simulink model "test_R2015b"  (R2015b)
settings: Solver=VariableStepAuto  StartTime=0.0  StopTime=10.0  RelTol=1e-3
settings Model: Creator=MiaoshunWu  LastModifiedBy=MiaoshunWu

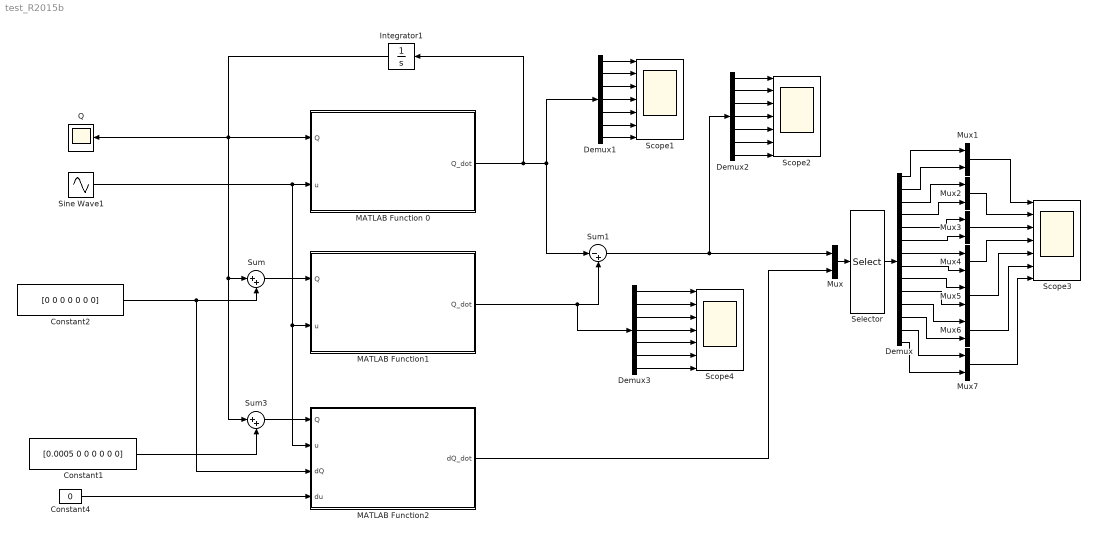
== system test_R2015b ==
  Constant1 : Constant  Value=[0.0005 0 0 0 0 0 0]
  Constant2 : Constant  Value=[0 0 0 0 0 0 0]
  Constant4 : Constant  Value=0
  Demux : Demux  Outputs=14
  Demux1 : Demux  Outputs=7
  Demux2 : Demux  Outputs=7
  Demux3 : Demux  Outputs=7
  Integrator1 : Integrator  InitialCondition=[0;0;0;0;0;0;0;]
  MATLAB Function 0 : MATLAB Function  TreatAsAtomicUnit=on
  MATLAB Function1 : MATLAB Function  TreatAsAtomicUnit=on
  MATLAB Function2 : MATLAB Function  TreatAsAtomicUnit=on
  Mux{,1..7} (8 alike) : Mux  Inputs=2
  Q : Scope
  Scope{1..4} (4 alike) : Scope  NumInputPorts=7
  Selector : Selector  InputPortWidth=14  IndexOptions=Index vector (dialog)  Indices=[1 8 2 9 3 10 4 11 5 12 6 13 7 14]  OutputSizes=1
  Sine Wave1 : Sin  SampleTime=0
  Sum : Sum  Inputs=|++
  Sum1 : Sum  Inputs=|-+
  Sum3 : Sum  Inputs=|++
  wires:
  MATLAB Function 0/1(Q_dot) -> Integrator1/1, Demux1/1, Sum1/1
  Sine Wave1/1 -> MATLAB Function 0/2(u), MATLAB Function1/2(u), MATLAB Function2/2(u)
  Sum/1 -> MATLAB Function1/1(Q)
  Integrator1/1 -> Sum3/1, Sum/1, Q/1, MATLAB Function 0/1(Q)
  MATLAB Function2/1(dQ_dot) -> Mux/2
  Constant2/1 -> MATLAB Function2/3(dQ), Sum/2
  Constant1/1 -> Sum3/2
  Sum3/1 -> MATLAB Function2/1(Q)
  Constant4/1 -> MATLAB Function2/4(du)
  Mux/1 -> Selector/1
  Selector/1 -> Demux/1
  Demux/1 -> Mux1/1
  Mux2/1 -> Scope3/2
  Mux3/1 -> Scope3/3
  Demux/7 -> Mux4/1
  Demux/8 -> Mux4/2
  Mux1/1 -> Scope3/1
  Mux4/1 -> Scope3/4
  Demux/6 -> Mux3/2
  Demux/5 -> Mux3/1
  Demux/4 -> Mux2/2
  Demux/3 -> Mux2/1
  Demux/2 -> Mux1/2
  Demux/9 -> Mux5/1
  Demux/10 -> Mux5/2
  Demux/11 -> Mux6/1
  Demux/12 -> Mux6/2
  Demux/13 -> Mux7/1
  Demux/14 -> Mux7/2
  Mux5/1 -> Scope3/5
  Mux6/1 -> Scope3/6
  Mux7/1 -> Scope3/7
  Demux1/1 -> Scope1/1
  Demux1/2 -> Scope1/2
  Demux1/3 -> Scope1/3
  Demux1/4 -> Scope1/4
  Demux1/5 -> Scope1/5
  Demux1/6 -> Scope1/6
  Demux1/7 -> Scope1/7
  Sum1/1 -> Demux2/1, Mux/1
  Demux2/1 -> Scope2/1
  Demux2/2 -> Scope2/2
  Demux2/3 -> Scope2/3
  Demux2/4 -> Scope2/4
  Demux2/5 -> Scope2/5
  Demux2/6 -> Scope2/6
  Demux2/7 -> Scope2/7
  MATLAB Function1/1(Q_dot) -> Demux3/1, Sum1/2
  Demux3/1 -> Scope4/1
  Demux3/2 -> Scope4/2
  Demux3/3 -> Scope4/3
  Demux3/4 -> Scope4/4
  Demux3/5 -> Scope4/5
  Demux3/6 -> Scope4/6
  Demux3/7 -> Scope4/7

== matlab function test_R2015b/MATLAB Function 0 ==
  data: Q_dot output; Q input; u input
function Q_dot  = DIP_Model(Q,u)
%{
%Description: Double inverted pendulum model
%Purpose: Simulates the double inverted pendulum through its mathematical 
%         dynamic model            
%Input Parameters: State space "Q", control input "u"
%Output Parameters: Derivative state space "Q_dot"
%Author: A. Arreortua
%**************************************************************************
%}
%% Definition of constants
% gravity acceleration
g = 9.81; % [m/s^2]
a1=0.085; %Distance between pivot and center of mass of pendulum1 [m]
a2=0.157; %Distance between pivot and center of mass of pendulum2 [m]
l1= 0.170; %Length of pendulum1 [m]
l2= 0.314;  %Length of pendulum2 [m]
m=0.5;  %Mass of the cart [kg]
m1=0.162; %Mass of pendulum1 [kg]
m2=0.203; %Mass of pendulum2 [kg]
J1 = (m1*l1^2)/12;    %Inertia of pendulum1 around the joint [kg m^2]
J2 = (m2*l2^2)/12;    %Inertia of pendulum2 around the joint [kg m^2]
% Model of motor behaviour: PT1 tau
T1 = 0.0395; % [s]
%Dinamic model constants
h1 = m+m1+m2;
h2 = m1*a1+m2*l1;
h3 = m2*a2;
h4 = m1*a1^2+m2*l1^2+J1;
h5 = m2*a2*l1;
h6 = m2*a2^2+J2;
h7 = m1*a1*g + m2*l1*g;
h8 = m2*a2*g;

%Q=[0;0;0;0;0;0];
det = (h4 * h6 - h5 * h5 * cos(Q(3) - Q(4)) * cos(Q(3) - Q(4)));
M11inv= [h6/det ,-h5*cos(Q(3)-Q(4))/det ; -h5*cos(Q(3)-Q(4))/det ,h4/det];
M11= [h6 ,-h5*cos(Q(3)-Q(4)) ; -h5*cos(Q(3)-Q(4)) ,h4];
M12 = [h2*cos(Q(3)); h3*cos(Q(4))];

C1 = [h5*(Q(2)^2)*sin(Q(3)-Q(4)); -h5*(Q(1)^2)*sin(Q(3)-Q(4))];
G1 = [-h7*sin(Q(3)); -h8*sin(Q(4))];
%% Dynamic equaations
x_2dot = u/T1- Q(6)/T1;  %%% x_2dot=
Theta_2dot = -M11inv*(M12* x_2dot + C1 + G1);
Q_dot = [Theta_2dot;Q(1);Q(2);Q(6);x_2dot;u*u];

== matlab function test_R2015b/MATLAB Function1 ==
  data: Q_dot output; Q input; u input
function Q_dot = DIP_Model(Q,u)
%% Definition of constants
% gravity acceleration
g = 9.81; % [m/s^2]
a1=0.085; %Distance between pivot and center of mass of pendulum1 [m]
a2=0.157; %Distance between pivot and center of mass of pendulum2 [m]
l1= 0.170; %Length of pendulum1 [m]
l2= 0.314;  %Length of pendulum2 [m]
m=0.5;  %Mass of the cart [kg]
m1=0.162; %Mass of pendulum1 [kg]
m2=0.203; %Mass of pendulum2 [kg]
J1 = (m1*l1^2)/12;    %Inertia of pendulum1 around the joint [kg m^2]
J2 = (m2*l2^2)/12;    %Inertia of pendulum2 around the joint [kg m^2]
% Model of motor behaviour: PT1 tau
T1 = 0.0395; % [s]
%Dinamic model constants
h1 = m+m1+m2;
h2 = m1*a1+m2*l1;
h3 = m2*a2;
h4 = m1*a1^2+m2*l1^2+J1;
h5 = m2*a2*l1;
h6 = m2*a2^2+J2;
h7 = m1*a1*g + m2*l1*g;
h8 = m2*a2*g;
%set up Q1-Q6
det = (h4*h6 - h5*h5*cos(Q(3)- Q(4)) * cos(Q(3)- Q(4)));
M11_inv= [h6/det ,-h5*cos(Q(3)-Q(4))/det ; -h5*cos(Q(3)-Q(4))/det ,h4/det];
M11= [h6 ,-h5*cos(Q(3)-Q(4)) ; -h5*cos(Q(3)-Q(4)) ,h4];
M12 = [h2*cos(Q(3)); h3*cos(Q(4))];

C1 = [h5*(Q(2)^2)*sin(Q(3)-Q(4)); -h5*(Q(1)^2)*sin(Q(3)-Q(4))];
G1 = [-h7*sin(Q(3)); -h8*sin(Q(4))];
% h7=h2*g
% double dx [7];
%Q(5)  =   dx(5)   / T1;
x_2dot = u/T1- Q(6)/T1; 
%x00 = -1 * M11_inv(1,1) *((x_2dot * M12(1)) + C1(1) + G1(1))+(-1) * M11_inv(1,2) * ((x_2dot * M12(1)) + C1(1) + G1(1));
x00 = -1 * M11_inv(1,1) * ((-1 *x_2dot * M12(1) ) + C1(1)+ G1(1))- M11_inv(1,2) * ((-1 * x_2dot * M12(1) ) + C1(2) + G1(2));%- ((M11_inv(1,1) * M12(1) + M11_inv(1,2) * M12(2))) / T1;
x01 = -1 * M11_inv(2,1) * ((-1 *x_2dot * M12(1) ) + C1(1)+ G1(1))- M11_inv(2,2) * ((-1 * x_2dot * M12(2) ) + C1(2) + G1(2));%- ((M11_inv(2,1) * M12(1) + M11_inv(2,2) * M12(2))) / T1;
%x01 = -1 * M11_inv(2,1) * ((x_2dot * M12(2)) + C1(2) + G1(2))+ (-1) * M11_inv(2,2) *( (x_2dot * M12(2)) + C1(2) + G1(2));
x02 = Q(1);
x03 = Q(2);
x04 = Q(6);
x05 =x_2dot ;
x06 = u * u;
Q_dot =[x00;x01;x02;x03;x04;x05;x06];
end

== matlab function test_R2015b/MATLAB Function2 ==
  data: dQ_dot output; Q input; u input; dQ input; du input
function dQ_dot  = DIP_Model(Q,u,dQ,du)
%{
%Description: Double inverted pendulum model
%Purpose: Simulates the double inverted pendulum through its mathematical 
%         dynamic model            
%Input Parameters: State space "Q", control input "u"
%Output Parameters: Derivative state space "Q_dot"
%Author: A. Arreortua
%**************************************************************************
%}
%% Definition of constants
% gravity acceleration
g = 9.81; % [m/s^2]
a1=0.085; %Distance between pivot and center of mass of pendulum1 [m]
a2=0.157; %Distance between pivot and center of mass of pendulum2 [m]
l1= 0.170; %Length of pendulum1 [m]
l2= 0.314;  %Length of pendulum2 [m]
m=0.5;  %Mass of the cart [kg]
m1=0.162; %Mass of pendulum1 [kg]
m2=0.203; %Mass of pendulum2 [kg]
J1 = (m1*l1^2)/12;    %Inertia of pendulum1 around the joint [kg m^2]
J2 = (m2*l2^2)/12;    %Inertia of pendulum2 around the joint [kg m^2]
% Model of motor behaviour: PT1 tau
T1 = 0.0395; % [s]
%Dinamic model constants
h1 = m+m1+m2;
h2 = m1*a1+m2*l1;
h3 = m2*a2;
h4 = m1*a1^2+m2*l1^2+J1;
h5 = m2*a2*l1;
h6 = m2*a2^2+J2;
h7 = m1*a1*g + m2*l1*g;
h8 = m2*a2*g;
%Q = [0;0;0;0;0;0];
%dQ= [0;0;0;0;0;0];
Q0=Q(1);
Q1=Q(2);
Q2=Q(3);
Q3=Q(4);
Q4=Q(5); 
Q5=Q(6); 


%//dQ0= -1 * M11_inv[0][0] * ((-1 * Q5 * M12[0] / T1) + C1[0] + G1[0]) - M11_inv[0][1] * ((-1 * Q5 * M12[1] / T1) + C1[1] + G1[1]) - (M11_inv[0][0] * M12[0] + M11_inv[0][1] * M12[1]) / T1;
s00 = -(2 * Q0 * h5 * h5 * cos(Q2 - Q3) * sin(Q2 - Q3)) / (h4 * h6 - h5 * h5 * cos(Q2 - Q3) * cos(Q2 - Q3));
s01= -(2 * Q1 * h5 * h6 * sin(Q2 - Q3)) / (h4 * h6 - h5 * h5 * cos(Q2 - Q3) * cos(Q2 - Q3));
s02= (h5 * sin(Q2 - Q3) * (h5 * sin(Q2 - Q3) * Q0 * Q0 + h8 * sin(Q3) + (Q5 * h3 * cos(Q2)) / T1)) / (h4 * h6 - h5 * h5 * cos(Q2 - Q3) * cos(Q2 - Q3)) - (h6 * (h5 * cos(Q2 - Q3) * Q1 * Q1 - h7 * cos(Q2) + (Q5 * h2 * sin(Q2)) / T1)) / (h4 * h6 - h5 * h5 * cos(Q2 - Q3) * cos(Q2 - Q3)) - (h5 * cos(Q2 - Q3) * (h5 * cos(Q2 - Q3) * Q0 * Q0 - (Q5 * h3 * sin(Q2)) / T1)) / (h4 * h6 - h5 * h5 * cos(Q2 - Q3) * cos(Q2 - Q3)) - u * ((h3 * h5 * cos(Q2) * sin(Q2 - Q3)) / (T1 * (h4 * h6 - h5 * h5 * cos(Q2 - Q3) * cos(Q2 - Q3))) - (h2 * h6 * sin(Q2)) / (T1 * (h4 * h6 - h5 * h5 * cos(Q2 - Q3) * cos(Q2 - Q3))) + (h3 * h5 * cos(Q2 - Q3) * sin(Q2)) / (T1 * (h4 * h6 - h5 * h5 * cos(Q2 - Q3) * cos(Q2 - Q3))) + (2 * h3 * h5 * h5 * h5 * cos(Q2) * cos(Q2 - Q3) * cos(Q2 - Q3) * sin(Q2 - Q3)) / (T1 * ((h4 * h6 - h5 * h5 * cos(Q2 - Q3) * cos(Q2 - Q3)) *(h4 * h6 - h5 * h5 * cos(Q2 - Q3) * cos(Q2 - Q3)))) - (2 * h2 * h5 * h5 * h6 * cos(Q2) * cos(Q2 - Q3) * sin(Q2 - Q3)) / (T1 * ((h4 * h6 - h5 * h5 * cos(Q2 - Q3) * cos(Q2 - Q3)) * (h4 * h6 - h5 * h5 * cos(Q2 - Q3) * cos(Q2 - Q3))))) + (2 * h5 * h5 * h5 * cos(Q2 - Q3) * cos(Q2 - Q3) * sin(Q2 - Q3) * (h5 * sin(Q2 - Q3) * Q0 * Q0 + h8 * sin(Q3) + (Q5 * h3 * cos(Q2)) / T1)) / ((h4 *h6 - h5 * h5 * cos(Q2 - Q3) * cos(Q2 - Q3)) * (h4 *h6 - h5 * h5 * cos(Q2 - Q3) * cos(Q2 - Q3))) - (2 * h5 * h5 * h6 * cos(Q2 - Q3) * sin(Q2 - Q3) * (-h5 * sin(Q2 - Q3) * Q1 * Q1 + h7 * sin(Q2) + (Q5 * h2 * cos(Q2)) / T1)) / ((h4 * h6 - h5 * h5 * cos(Q2 - Q3) * cos(Q2 - Q3)) * (h4 * h6 - h5 * h5 * cos(Q2 - Q3) * cos(Q2 - Q3)));
s03 =u * ((h3 * h5 * cos(Q2) * sin(Q2 - Q3)) / (T1 * (h4 * h6 - h5 * h5 * cos(Q2 - Q3) * cos(Q2 - Q3))) + (2 * h3 * h5 * h5 * h5 * cos(Q2) * cos(Q2 - Q3) * cos(Q2 - Q3) * sin(Q2 - Q3)) / (T1 * ((h4 * h6 - h5 * h5 * cos(Q2 - Q3) * cos(Q2 - Q3)) * (h4 * h6 - h5 * h5 * cos(Q2 - Q3) * cos(Q2 - Q3)))) - (2 * h2 * h5 * h5 * h6 * cos(Q2) * cos(Q2 - Q3) * sin(Q2 - Q3)) / (T1 * ((h4 * h6 - h5 * h5 * cos(Q2 - Q3) * cos(Q2 - Q3)) * (h4 * h6 - h5 * h5 * cos(Q2 - Q3) * cos(Q2 - Q3))))) - (h5 * sin(Q2 - Q3) * (h5 * sin(Q2 - Q3) * Q0 * Q0 + h8 * sin(Q3) + (Q5 * h3 * cos(Q2)) / T1)) / (h4 * h6 - h5 * h5 * cos(Q2 - Q3) * cos(Q2 - Q3)) - (h5 * cos(Q2 - Q3) * (-h5 * cos(Q2 - Q3) * Q0 * Q0 + h8 * cos(Q3))) / (h4 * h6 - h5 * h5 * cos(Q2 - Q3) * cos(Q2 - Q3)) - (2 * h5 * h5 * h5 * cos(Q2 - Q3) * cos(Q2 - Q3) * sin(Q2 - Q3) * (h5 * sin(Q2 - Q3) * Q0 * Q0 + h8 * sin(Q3) + (Q5 * h3 * cos(Q2)) / T1)) / ((h4 * h6 - h5 * h5 * cos(Q2 - Q3) * cos(Q2 - Q3)) * (h4 * h6 - h5 * h5 * cos(Q2 - Q3) * cos(Q2 - Q3))) + (Q1 * Q1 * h5 * h6 * cos(Q2 - Q3)) / (h4 * h6 - h5 * h5 * cos(Q2 - Q3) * cos(Q2 - Q3)) + (2 * h5 * h5 * h6 * cos(Q2 - Q3) * sin(Q2 - Q3) * (-h5 * sin(Q2 - Q3) * Q1 * Q1 + h7 * sin(Q2) + (Q5 * h2 * cos(Q2)) / T1)) / ((h4 * h6 - h5 * h5 * cos(Q2 - Q3) * cos(Q2 - Q3)) * (h4 * h6 - h5 * h5 * cos(Q2 - Q3) * cos(Q2 - Q3)));
s04 = 0;
s05 = (h2 * h6 * cos(Q2)+h3 * h5 * cos(Q3) * cos(Q2 - Q3)) / (T1 * (h4 * h6 - h5 * h5 * cos(Q2 - Q3) * cos(Q2 - Q3)));
s06 = (h3 * h5 * cos(Q2) * cos(Q2 - Q3)) / (T1 * (h4 * h6 - h5 * h5 * cos(Q2 - Q3) * cos(Q2 - Q3))) - (h2 * h6 * cos(Q2)) / (T1 * (h4 * h6 - h5 * h5 * cos(Q2 - Q3) * cos(Q2 - Q3)));
ddQ0 = dQ(1)*s00+dQ(2)*s01+dQ(3)*s02+dQ(4)*s03+dQ(5)*s04+dQ(6)*s05+du*s06



s10 = (2 * Q0 * h4 * h5 * sin(Q2 - Q3)) / (h4 * h6 - h5 * h5 * cos(Q2 - Q3) * cos(Q2 - Q3));
s11 = (2 * Q1 * h5 * h5 * cos(Q2 - Q3) * sin(Q2 - Q3)) / (h4 * h6 - h5 * h5 * cos(Q2 - Q3) * cos(Q2 - Q3));
s12= (h4 * (h5 * cos(Q2 - Q3) * Q0 * Q0 - (Q5 * h3 * sin(Q2)) / T1)) / (h4 * h6 - h5 * h5 * cos(Q2 - Q3) * cos(Q2 - Q3)) - u * ((h2 * h5 * cos(Q2) * sin(Q2 - Q3)) / (T1 * (h4 * h6 - h5 * h5 * cos(Q2 - Q3) * cos(Q2 - Q3))) - (h3 * h4 * sin(Q2)) / (T1 * (h4 * h6 - h5 * h5 * cos(Q2 - Q3) * cos(Q2 - Q3))) + (h2 * h5 * cos(Q2 - Q3) * sin(Q2)) / (T1 * (h4 * h6 - h5 * h5 * cos(Q2 - Q3) * cos(Q2 - Q3))) + (2 * h2 * h5 * h5 * h5 * cos(Q2) * cos(Q2 - Q3) * cos(Q2 - Q3) * sin(Q2 - Q3)) / (T1 * ((h4 * h6 - h5 * h5 * cos(Q2 - Q3) * cos(Q2 - Q3)) * (h4 * h6 - h5 * h5 * cos(Q2 - Q3) * cos(Q2 - Q3)))) - (2 * h3 * h4 * h5 * h5 * cos(Q2) * cos(Q2 - Q3) * sin(Q2 - Q3)) / (T1 * ((h4 * h6 - h5 * h5 * cos(Q2 - Q3) * cos(Q2 - Q3)) * (h4 * h6 - h5 * h5 * cos(Q2 - Q3) * cos(Q2 - Q3))))) + (h5 * cos(Q2 - Q3) * (h5 * cos(Q2 - Q3) * Q1 * Q1 - h7 * cos(Q2) + (Q5 * h2 * sin(Q2)) / T1)) / (h4 * h6 - h5 * h5 * cos(Q2 - Q3) * cos(Q2 - Q3)) + (h5 * sin(Q2 - Q3) * (-h5 * sin(Q2 - Q3) * Q1 * Q1 + h7 * sin(Q2) + (Q5 * h2 * cos(Q2)) / T1)) / (h4 * h6 - h5 * h5 * cos(Q2 - Q3) * cos(Q2 - Q3)) + (2 * h5 * h5 * h5 * cos(Q2 - Q3) * cos(Q2 - Q3) * sin(Q2 - Q3) * (-h5 * sin(Q2 - Q3) * Q1 * Q1 + h7 * sin(Q2) + (Q5 * h2 * cos(Q2)) / T1)) / ((h4 * h6 - h5 * h5 * cos(Q2 - Q3) * cos(Q2 - Q3)) * (h4 * h6 - h5 * h5 * cos(Q2 - Q3) * cos(Q2 - Q3))) - (2 * h4 * h5 * h5 * cos(Q2 - Q3) * sin(Q2 - Q3) * (h5 * sin(Q2 - Q3) * Q0 * Q0 + h8 * sin(Q3) + (Q5 * h3 * cos(Q2)) / T1)) / ((h4 * h6 - h5 * h5 * cos(Q2 - Q3) * cos(Q2 - Q3)) * (h4 * h6 - h5 * h5 * cos(Q2 - Q3) * cos(Q2 - Q3)));
s13 = u * ((h2 * h5 * cos(Q2) * sin(Q2 - Q3)) / (T1 * (h4 * h6 - h5 * h5 * cos(Q2 - Q3) * cos(Q2 - Q3))) + (2 * h2 * h5 * h5 * h5 * cos(Q2) * cos(Q2 - Q3) * cos(Q2 - Q3) * sin(Q2 - Q3)) / (T1 * ((h4 * h6 - h5 * h5 * cos(Q2 - Q3) * cos(Q2 - Q3)) * (h4 * h6 - h5 * h5 * cos(Q2 - Q3) * cos(Q2 - Q3)))) - (2 * h3 * h4 * h5 * h5 * cos(Q2) * cos(Q2 - Q3) * sin(Q2 - Q3)) / (T1 * ((h4 * h6 - h5 * h5 * cos(Q2 - Q3) * cos(Q2 - Q3)) * (h4 * h6 - h5 * h5 * cos(Q2 - Q3) * cos(Q2 - Q3))))) + (h4 * (-h5 * cos(Q2 - Q3) * Q0 * Q0 + h8 * cos(Q3))) / (h4 * h6 - h5 * h5 * cos(Q2 - Q3) * cos(Q2 - Q3)) - (Q1 * Q1 * h5 * h5 * cos(Q2 - Q3) * cos(Q2 - Q3)) / (h4 * h6 - h5 * h5 * cos(Q2 - Q3) * cos(Q2 - Q3)) - (h5 * sin(Q2 - Q3) * (-h5 * sin(Q2 - Q3) * Q1 * Q1 + h7 * sin(Q2) + (Q5 * h2 * cos(Q2)) / T1)) / (h4 * h6 - h5 * h5 * cos(Q2 - Q3) * cos(Q2 - Q3)) - (2 * h5 * h5 * h5 * cos(Q2 - Q3) * cos(Q2 - Q3) * sin(Q2 - Q3) * (-h5 * sin(Q2 - Q3) * Q1 * Q1 + h7 * sin(Q2) + (Q5 * h2 * cos(Q2)) / T1)) / ((h4 * h6 - h5 * h5 * cos(Q2 - Q3) * cos(Q2 - Q3)) * (h4 * h6 - h5 * h5 * cos(Q2 - Q3) * cos(Q2 - Q3))) + (2 * h4 * h5 * h5 * cos(Q2 - Q3) * sin(Q2 - Q3) * (h5 * sin(Q2 - Q3) * Q0 * Q0 + h8 * sin(Q3) + (Q5 * h3 * cos(Q2)) / T1)) / ((h4 * h6 - h5 * h5 * cos(Q2 - Q3) * cos(Q2 - Q3)) * (h4 * h6 - h5 * h5 * cos(Q2 - Q3) * cos(Q2 - Q3)));
s14 = 0;
s15 =  ((h3 * h4 * cos(Q3)) - (h2 * h5 * cos(Q2) * cos(Q2 - Q3))) / (T1 * (h4 * h6 - h5 * h5 * cos(Q2 - Q3) * cos(Q2 - Q3)));
s16 = (h2 * h5 * cos(Q2) * cos(Q2 - Q3)) / (T1 * (h4 * h6 - h5 * h5 * cos(Q2 - Q3) * cos(Q2 - Q3))) - (h3 * h4 * cos(Q2)) / (T1 * (h4 * h6 - h5 * h5 * cos(Q2 - Q3) * cos(Q2 - Q3)));


ddQ1=dQ(1)*s10+dQ(2)*s11+dQ(3)*s12+dQ(4)*s13+dQ(5)*s14+dQ(6)*s15+du*s16

ddQ2=s10;
%s(2, x_indexode(0)) = 1;
%s(2, x_indexode(1)) = 0;
%s(2, x_indexode(2)) = 0;
%s(2, x_indexode(3)) = 0;
%s(2, x_indexode(4)) = 0;
%s(2, x_indexode(5)) = 0;
%s(2, u_indexode(0)) = 0;

ddQ3=dQ(2);
%s(3, x_indexode(0)) = 0;
%s(3, x_indexode(1)) = 1;
%s(3, x_indexode(2)) = 0;
%s(3, x_indexode(3)) = 0;
%s(3, x_indexode(4)) = 0;
%s(3, x_indexode(5)) = 0;
%s(3, u_indexode(0)) = 0;

 ddQ4=dQ(6);
%s(4, x_indexode(0)) = 0;
%s(4, x_indexode(1)) = 0;
%s(4, x_indexode(2)) = 0;
%s(4, x_indexode(3)) = 0;
%s(4, x_indexode(4)) = 0;
%s(4, x_indexode(5)) = 1;
%s(4, u_indexode(0)) = 0;

 ddQ5=-1 * (dQ(6) - du) / T1;
%s(5, x_indexode(0)) = 0;
%s(5, x_indexode(1)) = 0;
%s(5, x_indexode(2)) = 0;
%s(5, x_indexode(3)) = 0;
%s(5, x_indexode(4)) = 0;
%s(5, x_indexode(5)) = -1 / T1;
%s(5, u_indexode(0)) = 1 / T1;
 ddQ6 =(du * du);
%s(6, x_indexode(0)) = 0;     //!!!!!
%s(6, x_indexode(1)) = 0;
%s(6, x_indexode(2)) = 0;
%s(6, x_indexode(3)) = 0;
%s(6, x_indexode(4)) = 0;
%s(6, x_indexode(5)) = 0;
%s(6, u_indexode(0)) = 2 * u;

%% Dynamic equations
dQ_dot=[ddQ0;ddQ1;ddQ2;ddQ3;ddQ4;ddQ5;ddQ6];
